simulink model "voter_circuit"  (R2018b)
settings: Solver=VariableStepAuto  StartTime=0.0  StopTime=10.0  RelTol=1e-3
settings Model: Creator=hiterd  LastModifiedBy=hiterd

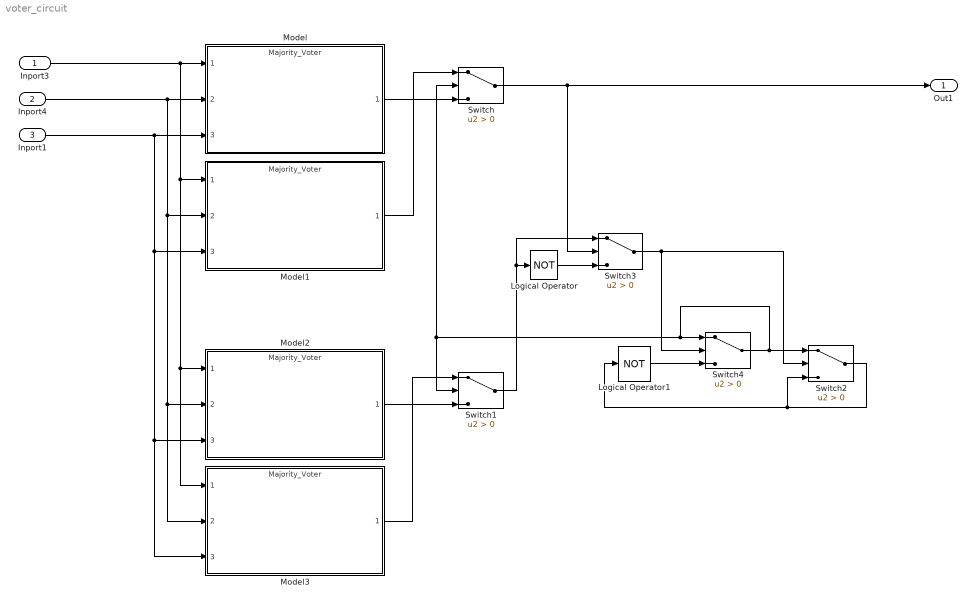
== system voter_circuit ==
  Inport3 : Inport
  Inport4 : Inport  Port=2
  Inport1 : Inport  Port=3
  Logical Operator : Logic  Operator=NOT  IconShape=distinctive  AllPortsSameDT=off  OutDataTypeStr=boolean
  Logical Operator1 : Logic  Operator=NOT  IconShape=distinctive  AllPortsSameDT=off  OutDataTypeStr=boolean
  Model{,1..3} (4 alike) : ModelReference  ModelNameDialog=Majority_Voter.slx  SimulationMode=Normal  ModelReferenceVersion=1.3
  Switch{,1..4} (5 alike) : Switch  Criteria=u2 > Threshold
  Out1 : Outport
  wires:
  Inport3/1 -> Model1/1, Model2/1, Model3/1, Model/1
  Inport4/1 -> Model1/2, Model2/2, Model3/2, Model/2
  Inport1/1 -> Model1/3, Model2/3, Model3/3, Model/3
  Model1/1 -> Switch/1
  Model/1 -> Switch/3
  Model2/1 -> Switch1/3
  Model3/1 -> Switch1/1
  Switch/1 -> Out1/1, Switch3/2
  Switch3/1 -> Switch2/2, Switch4/2
  Switch4/1 -> Switch4/1, Switch1/2, Switch/2, Switch2/1
  Logical Operator/1 -> Switch3/3
  Logical Operator1/1 -> Switch4/3
  Switch2/1 -> Switch2/3, Logical Operator1/1
  Switch1/1 -> Logical Operator/1, Switch3/1
